simulink library "xpcseriallib"  (Simulink 7.7)
settings: Solver=FixedStepDiscrete  StartTime=0.0  StopTime=inf  RelTol=1e-3
undefined symbols (not defined in the file or in its folder): baddr1, baddr2, mbaseserialbinmask, mbaseserialmask, mdiamondemeraldfifomask, mdiamondemeraldmask, mmodemcontrol, mqua2mask, mquafifomask, mquamask, mrs232
libraries: xpcseriallib x614, xpclib x16, simulink x12
(part 4 of 7)

== system xpcseriallib/Diamond/Emerald-MM /Diamond Emerald-MM ==
  "Enable TX " : S-Function  FunctionName=sertxenableemeraldmm  Parameters=addr  EnableBusSupport=off  mask(Enable TX Int){addr=-1}
      mask prompts: addr "Base address:"
      mask help:
      | Diamond Emerald
      | Enable TX Interrupt
      mask init:
      | addr = hex2dec( addr(3:end) );
      mask Help: helpview(fullfile(docroot, 'mapfiles', 'xpc.map'), 'Baseboard_Enable_Int')
      mask Display:
      | disp('Diamond\nEmerald-MM\nEnable TX int');
      | port_label('input', 1, 'E');
  Filter Int Reason : S-Function  FunctionName=filterserint  Parameters=port, value  EnableBusSupport=off  mask(Interrupt Source Filter){port=1, value=Receive data}
      mask prompts: value "Filter value:"
      mask help:
      | Diamond Emerald-MM
      | Interrupt Source Filter
      mask Help: helpview(fullfile(docroot, 'mapfiles', 'xpc.map'), 'Baseboard_Filter_Ints')
      mask StyleString: popup(1|2|3|4),popup(Receive data|Transmitter empty|Modem status change)
      mask Display:
      | disp('Diamond\nEmerald\nFilter');
      | port_label('input', 1, 'S' );
      | port_label('output', 1, 'E' );
  Read HW FIFO : S-Function  FunctionName=serreademeraldmm  Parameters=addr, flush  EnableBusSupport=off  mask(Read Data Port){flush=on, addr=0}
      mask prompts: flush "Flush HW FIFO on startup"; addr "Base address:"
      mask help:
      | Diamond Emerald-MM
      | Read Data Port
      mask init:
      | addr = hex2dec( addr(3:end) );
      mask Help: helpview(fullfile(docroot, 'mapfiles', 'xpc.map'), 'Baseboard_Read_HW')
      mask Display:
      | disp('Diamond\nEmerald-MM\nRead Data Port');
      | port_label('input', 1, 'E');
      | port_label('output', 1, 'D');
  Read Int Status : S-Function  FunctionName=iqueryemeraldmm  Parameters=addr1, addr2, addr3, addr4, intstat  EnableBusSupport=off  mask(Interrupt Query){addr1=0, addr2=0, addr3=0, addr4=0, intstat=0}
      mask prompts: addr1 "First port address:"; addr2 "Second port address:"; addr3 "Third port address:"; addr4 "Fourth port address:"; intstat "Interrupt status address"
      mask help:
      | Diamond Emerald-MM
      | Interrupt Query
      mask init:
      | addr1 = hex2dec( addr1(3:end) );
      | addr2 = hex2dec( addr2(3:end) );
      | addr3 = hex2dec( addr3(3:end) );
      | addr4 = hex2dec( addr4(3:end) );
      | intstat = hex2dec( intstat(3:end) );
      mask Help: helpview(fullfile(docroot, 'mapfiles', 'xpc.map'), 'Baseboard_Interrupt_Query')
      mask Display:
      | disp('Diamond\nEmerald-MM\nInt Status');
      | port_label('output', 1, 'S' );
  Setup : S-Function  FunctionName=sersetupemeraldmm  Parameters=addr, baud, width, nstop, parity, fmode, ctsmode, rlevel  EnableBusSupport=off  mask(setup){baud=115200  (HS 460800), width=8, nstop=1, parity=None, fmode=16 deep, rlevel=half full, ctsmode=on, addr=0}
      mask prompts: baud "Baud rate:"; width "Number of data bits:"; nstop "Number of stop bits:"; fmode "FIFO mode:"; rlevel "Receive trigger level:"; ctsmode "Enable auto RTS/CTS"; addr "Base address:"
      mask help:
      | Diamond Emerald-MM
      | Serial
      | Setup
      mask init:
      | addr = hex2dec( addr(3:end) );
      mask Help: helpview(fullfile(docroot, 'mapfiles', 'xpc.map'), 'Baseboard_Setup')
      mask StyleString: popup(115200  (HS 460800)|57600   (HS 230400)|38400   (HS 153600)|28800   (HS 115200)|19200   (HS 76800)|14400   (HS 57600)|9600    (HS 38400)|4800    (HS 19200)|2400    (HS 9600)|1200    (HS 4800)|600     (HS 2400)|300     (HS 1200)|150     (HS 600)|110     (HS 440)|75      (HS 300)|27.5    (HS 110)),popup(5|6|7|8),popup(1|2),popup(None|Even|Odd|Mark|Space),popup(64 deep|16 deep|1 deep),popup(1|quarter full|half full|almost full),checkbox,edit
      mask Display: disp('Diamond\nEmerald-MM\nSetup');
  Write HW FIFO : S-Function  FunctionName=serwriteemeraldmm  Parameters=addr  EnableBusSupport=off  mask(Write Data Port){addr=-1}
      mask prompts: addr "Base address:"
      mask help:
      | Diamond Emerald-MM
      | Write Data Port
      mask init:
      | addr = hex2dec( addr(3:end) );
      mask Help: helpview(fullfile(docroot, 'mapfiles', 'xpc.map'), 'Baseboard_Write_HW')
      mask Display:
      | disp('Diamond\nEmerald-MM\nWrite Data Port');
      | port_label('input', 1, 'D');
      | port_label('input', 2, 'E');

== system xpcseriallib/Diamond/Emerald-MM /Diamond Emerald-MM Serial ==
  In1 : Inport
  In2 : Inport  Port=2
  In3 : Inport  Port=3
  In4 : Inport  Port=4
  Enable TX 1 : xpcseriallib/Diamond/Emerald-MM /Diamond Emerald-MM/Enable TX   addr=baddr1
  Enable TX 2 : xpcseriallib/Diamond/Emerald-MM /Diamond Emerald-MM/Enable TX   addr=baddr2
  Enable TX 3 : xpcseriallib/Diamond/Emerald-MM /Diamond Emerald-MM/Enable TX   addr=baddr3
  Enable TX 4 : xpcseriallib/Diamond/Emerald-MM /Diamond Emerald-MM/Enable TX   addr=baddr4
  FIFO read {1..4} (4 alike) : xpcseriallib/FIFO read   maxsize=1024  minsize=1  usedelimiter=on  delimiter=13  outputtype=count+16 bit uint  enable=off  enableout=off  sampletime=-1
  FIFO write 1 : xpcseriallib/FIFO write   size=1024  inputtype=8 bit uint null terminated  present=on  sampletime=-1  id=XMT channel 1, IRQ 7
  FIFO write 2 : xpcseriallib/FIFO write   size=1024  inputtype=8 bit uint null terminated  present=on  sampletime=-1  id=XMT channel 2, IRQ 7
  FIFO write 3 : xpcseriallib/FIFO write   size=1024  inputtype=8 bit uint null terminated  present=on  sampletime=-1  id=XMT channel 3, IRQ 7
  FIFO write 4 : xpcseriallib/FIFO write   size=1024  inputtype=8 bit uint null terminated  present=on  sampletime=-1  id=XMT channel 4, IRQ 7
  IRQ Source : xpclib/Asynchronous Event/IRQ Source  irqNo=7  preempt=10  b_type=None/Other  slot=-1
  RS232 ISR : Subsystem  TreatAsAtomicUnit=on  mask(RS232 ISR){addr1=baddr1, addr2=baddr2, addr3=baddr3, addr4=baddr4, intstat=istat}
      mask prompts: addr1 "First channel address:"; addr2 "Second channel address:"; addr3 "Third channel address:"; addr4 "Fourth channel address:"; intstat "Status register address:"
      mask help:
      | Baseboard Serial
      | Interrupt Service Routine
      mask init:
      | baddr1 = addr1;
      | baddr2 = addr2;
      | baddr3 = addr3;
      | baddr4 = addr4;
      | istat = intstat;
      mask Display:
      | disp('Diamond\nEmerald\nSerial\nISR');
      | port_label('input', 1, 'XMT1');
      | port_label('input', 2, 'XMT2');
      | port_label('input', 3, 'XMT3');
      | port_label('input', 4, 'XMT4');
      | port_label('output', 1, 'RCV1');
      | port_label('output', 2, 'RCV2');
      | port_label('output', 3, 'RCV3');
      | port_label('output', 4, 'RCV4');
  Rate Transition{,1..7} (8 alike) : RateTransition  Integrity=off  Deterministic=off
  Setup1 : xpcseriallib/Diamond/Emerald-MM /Diamond Emerald-MM/Setup  baud="115200  (HS 460800)"  width=8  nstop=1  parity=None  fmode=16 deep  rlevel=half full  ctsmode=on  addr=baddr1
  Setup2 : xpcseriallib/Diamond/Emerald-MM /Diamond Emerald-MM/Setup  baud="115200  (HS 460800)"  width=8  nstop=1  parity=None  fmode=16 deep  rlevel=half full  ctsmode=on  addr=baddr2
  Setup3 : xpcseriallib/Diamond/Emerald-MM /Diamond Emerald-MM/Setup  baud="115200  (HS 460800)"  width=8  nstop=1  parity=None  fmode=16 deep  rlevel=half full  ctsmode=on  addr=baddr3
  Setup4 : xpcseriallib/Diamond/Emerald-MM /Diamond Emerald-MM/Setup  baud="115200  (HS 460800)"  width=8  nstop=1  parity=None  fmode=16 deep  rlevel=half full  ctsmode=on  addr=baddr4
  Out1 : Outport
  Out2 : Outport  Port=2
  Out3 : Outport  Port=3
  Out4 : Outport  Port=4
  wires:
  FIFO write 1/2 -> Enable TX 1/1
  IRQ Source/1 -> RS232 ISR/Trigger
  Rate Transition/1 -> RS232 ISR/1(Xmt 1)
  FIFO write 1/1 -> Rate Transition/1
  In1/1 -> FIFO write 1/1
  FIFO write 2/1 -> Rate Transition2/1
  In2/1 -> FIFO write 2/1
  Rate Transition1/1 -> FIFO read 1/1
  FIFO read 1/1 -> Out1/1
  Rate Transition3/1 -> FIFO read 2/1
  FIFO read 2/1 -> Out2/1
  RS232 ISR/1(Recv 1) -> Rate Transition1/1
  RS232 ISR/2(Recv 2) -> Rate Transition3/1
  Rate Transition2/1 -> RS232 ISR/2(Xmt 2)
  In4/1 -> FIFO write 4/1
  In3/1 -> FIFO write 3/1
  FIFO read 3/1 -> Out3/1
  FIFO read 4/1 -> Out4/1
  Rate Transition5/1 -> FIFO read 3/1
  Rate Transition7/1 -> FIFO read 4/1
  FIFO write 4/1 -> Rate Transition6/1
  FIFO write 3/1 -> Rate Transition4/1
  Rate Transition4/1 -> RS232 ISR/3(Xmt 3)
  Rate Transition6/1 -> RS232 ISR/4(Xmt 4)
  RS232 ISR/3(Recv 3) -> Rate Transition5/1
  RS232 ISR/4(Recv 4) -> Rate Transition7/1
  FIFO write 2/2 -> Enable TX 2/1
  FIFO write 3/2 -> Enable TX 3/1
  FIFO write 4/2 -> Enable TX 4/1

== system xpcseriallib/Diamond/Emerald-MM /Diamond Emerald-MM Serial F ==
  In1 : Inport
  In2 : Inport  Port=2
  In3 : Inport  Port=3
  In4 : Inport  Port=4
  Enable TX 1 : xpcseriallib/Diamond/Emerald-MM /Diamond Emerald-MM/Enable TX   addr=baddr1
  Enable TX 2 : xpcseriallib/Diamond/Emerald-MM /Diamond Emerald-MM/Enable TX   addr=baddr2
  Enable TX 3 : xpcseriallib/Diamond/Emerald-MM /Diamond Emerald-MM/Enable TX   addr=baddr3
  Enable TX 4 : xpcseriallib/Diamond/Emerald-MM /Diamond Emerald-MM/Enable TX   addr=baddr4
  FIFO write 1 : xpcseriallib/FIFO write   size=1024  inputtype=8 bit uint null terminated  present=on  sampletime=-1  id=XMT channel 1, IRQ 7
  FIFO write 2 : xpcseriallib/FIFO write   size=1024  inputtype=8 bit uint null terminated  present=on  sampletime=-1  id=XMT channel 2, IRQ 7
  FIFO write 3 : xpcseriallib/FIFO write   size=1024  inputtype=8 bit uint null terminated  present=on  sampletime=-1  id=XMT channel 3, IRQ 7
  FIFO write 4 : xpcseriallib/FIFO write   size=1024  inputtype=8 bit uint null terminated  present=on  sampletime=-1  id=XMT channel 4, IRQ 7
  IRQ Source : xpclib/Asynchronous Event/IRQ Source  irqNo=7  preempt=10  b_type=None/Other  slot=-1
  RS232 ISR : Subsystem  TreatAsAtomicUnit=on  mask(RS232 ISR){addr1=baddr1, addr2=baddr2, addr3=baddr3, addr4=baddr4, intstat=istat}
      mask prompts: addr1 "First channel address:"; addr2 "Second channel address:"; addr3 "Third channel address:"; addr4 "Fourth channel address:"; intstat "Status register address:"
      mask help:
      | Baseboard Serial
      | Interrupt Service Routine
      mask init:
      | baddr1 = addr1;
      | baddr2 = addr2;
      | baddr3 = addr3;
      | baddr4 = addr4;
      | istat = intstat;
      mask Display:
      | disp('Diamond\nEmerald\nSerial\nISR');
      | port_label('input', 1, 'XMT1');
      | port_label('input', 2, 'XMT2');
      | port_label('input', 3, 'XMT3');
      | port_label('input', 4, 'XMT4');
      | port_label('output', 1, 'RCV1');
      | port_label('output', 2, 'RCV2');
      | port_label('output', 3, 'RCV3');
      | port_label('output', 4, 'RCV4');
  Rate Transition{,2,4,6} (4 alike) : RateTransition  Integrity=off  Deterministic=off
  Rate Transition{1,3,5,7} (4 alike) : RateTransition  Integrity=off  Deterministic=off  OutPortSampleTime=0
  Setup1 : xpcseriallib/Diamond/Emerald-MM /Diamond Emerald-MM/Setup  baud="115200  (HS 460800)"  width=8  nstop=1  parity=None  fmode=16 deep  rlevel=half full  ctsmode=on  addr=baddr1
  Setup2 : xpcseriallib/Diamond/Emerald-MM /Diamond Emerald-MM/Setup  baud="115200  (HS 460800)"  width=8  nstop=1  parity=None  fmode=16 deep  rlevel=half full  ctsmode=on  addr=baddr2
  Setup3 : xpcseriallib/Diamond/Emerald-MM /Diamond Emerald-MM/Setup  baud="115200  (HS 460800)"  width=8  nstop=1  parity=None  fmode=16 deep  rlevel=half full  ctsmode=on  addr=baddr3
  Setup4 : xpcseriallib/Diamond/Emerald-MM /Diamond Emerald-MM/Setup  baud="115200  (HS 460800)"  width=8  nstop=1  parity=None  fmode=16 deep  rlevel=half full  ctsmode=on  addr=baddr4
  Out1 : Outport
  Out2 : Outport  Port=2
  Out3 : Outport  Port=3
  Out4 : Outport  Port=4
  wires:
  FIFO write 1/2 -> Enable TX 1/1
  IRQ Source/1 -> RS232 ISR/Trigger
  Rate Transition/1 -> RS232 ISR/1(Xmt 1)
  FIFO write 1/1 -> Rate Transition/1
  In1/1 -> FIFO write 1/1
  FIFO write 2/1 -> Rate Transition2/1
  In2/1 -> FIFO write 2/1
  Rate Transition1/1 -> Out1/1
  Rate Transition3/1 -> Out2/1
  RS232 ISR/1(Recv 1) -> Rate Transition1/1
  RS232 ISR/2(Recv 2) -> Rate Transition3/1
  Rate Transition2/1 -> RS232 ISR/2(Xmt 2)
  In4/1 -> FIFO write 4/1
  In3/1 -> FIFO write 3/1
  Rate Transition5/1 -> Out3/1
  Rate Transition7/1 -> Out4/1
  FIFO write 4/1 -> Rate Transition6/1
  FIFO write 3/1 -> Rate Transition4/1
  Rate Transition4/1 -> RS232 ISR/3(Xmt 3)
  Rate Transition6/1 -> RS232 ISR/4(Xmt 4)
  RS232 ISR/3(Recv 3) -> Rate Transition5/1
  RS232 ISR/4(Recv 4) -> Rate Transition7/1
  FIFO write 2/2 -> Enable TX 2/1
  FIFO write 3/2 -> Enable TX 3/1
  FIFO write 4/2 -> Enable TX 4/1

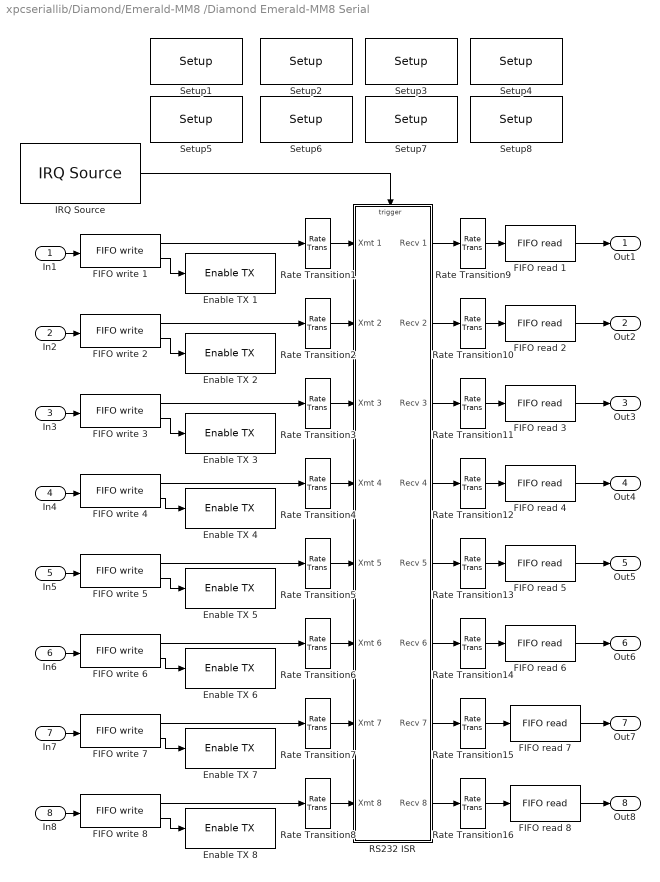
== system xpcseriallib/Diamond/Emerald-MM8 /Diamond Emerald-MM8 Serial ==
  In1 : Inport
  In2 : Inport  Port=2
  In3 : Inport  Port=3
  In4 : Inport  Port=4
  In5 : Inport  Port=5
  In6 : Inport  Port=6
  In7 : Inport  Port=7
  In8 : Inport  Port=8
  Enable TX 1 : xpcseriallib/Diamond/Emerald-MM8 /Diamond Emerald-MM8 /Enable TX   addr=baddr1
  Enable TX 2 : xpcseriallib/Diamond/Emerald-MM8 /Diamond Emerald-MM8 /Enable TX   addr=baddr2
  Enable TX 3 : xpcseriallib/Diamond/Emerald-MM8 /Diamond Emerald-MM8 /Enable TX   addr=baddr3
  Enable TX 4 : xpcseriallib/Diamond/Emerald-MM8 /Diamond Emerald-MM8 /Enable TX   addr=baddr4
  Enable TX 5 : xpcseriallib/Diamond/Emerald-MM8 /Diamond Emerald-MM8 /Enable TX   addr=baddr5
  Enable TX 6 : xpcseriallib/Diamond/Emerald-MM8 /Diamond Emerald-MM8 /Enable TX   addr=baddr6
  Enable TX 7 : xpcseriallib/Diamond/Emerald-MM8 /Diamond Emerald-MM8 /Enable TX   addr=baddr7
  Enable TX 8 : xpcseriallib/Diamond/Emerald-MM8 /Diamond Emerald-MM8 /Enable TX   addr=baddr8
  FIFO read {1..8} (8 alike) : xpcseriallib/FIFO read   maxsize=1024  minsize=1  usedelimiter=on  delimiter=13  outputtype=count+16 bit uint  enable=off  enableout=off  sampletime=-1
  FIFO write 1 : xpcseriallib/FIFO write   size=1024  inputtype=8 bit uint null terminated  present=on  sampletime=-1  id=XMT channel 1, IRQ 5
  FIFO write 2 : xpcseriallib/FIFO write   size=1024  inputtype=8 bit uint null terminated  present=on  sampletime=-1  id=XMT channel 2, IRQ 5
  FIFO write 3 : xpcseriallib/FIFO write   size=1024  inputtype=8 bit uint null terminated  present=on  sampletime=-1  id=XMT channel 3, IRQ 5
  FIFO write 4 : xpcseriallib/FIFO write   size=1024  inputtype=8 bit uint null terminated  present=on  sampletime=-1  id=XMT channel 4, IRQ 5
  FIFO write 5 : xpcseriallib/FIFO write   size=1024  inputtype=8 bit uint null terminated  present=on  sampletime=-1  id=XMT channel 5, IRQ 5
  FIFO write 6 : xpcseriallib/FIFO write   size=1024  inputtype=8 bit uint null terminated  present=on  sampletime=-1  id=XMT channel 6, IRQ 5
  FIFO write 7 : xpcseriallib/FIFO write   size=1024  inputtype=8 bit uint null terminated  present=on  sampletime=-1  id=XMT channel 7, IRQ 5
  FIFO write 8 : xpcseriallib/FIFO write   size=1024  inputtype=8 bit uint null terminated  present=on  sampletime=-1  id=XMT channel 8, IRQ 5
  IRQ Source : xpclib/Asynchronous Event/IRQ Source  irqNo=5  preempt=10  b_type=None/Other  slot=-1
  RS232 ISR : Subsystem  TreatAsAtomicUnit=on  mask(RS232 ISR){addr1=baddr1, addr2=baddr2, addr3=baddr3, addr4=baddr4, intstat=istat}
      mask prompts: addr1 "First channel address:"; addr2 "Second channel address:"; addr3 "Third channel address:"; addr4 "Fourth channel address:"; intstat "Status register address:"
      mask help:
      | Baseboard Serial
      | Interrupt Service Routine
      mask init:
      | baddr1 = addr1;
      | baddr2 = addr2;
      | baddr3 = addr3;
      | baddr4 = addr4;
      | istat = intstat;
      mask Display:
      | disp('Diamond\nEmerald\nSerial\nISR');
      | port_label('input', 1, 'XMT1');
      | port_label('input', 2, 'XMT2');
      | port_label('input', 3, 'XMT3');
      | port_label('input', 4, 'XMT4');
      | port_label('input', 5, 'XMT5');
      | port_label('input', 6, 'XMT6');
      | port_label('input', 7, 'XMT7');
      | port_label('input', 8, 'XMT8');
      | port_label('output', 1, 'RCV1');
      | port_label('output', 2, 'RCV2');
      | port_label('output', 3, 'RCV3');
      | port_label('output', 4, 'RCV4');
      | port_label('output', 5, 'RCV5');
      | port_label('output', 6, 'RCV6');
      | port_label('output', 7, 'RCV7');
      | port_label('output', 8, 'RCV8');
  Rate Transition{1..16} (16 alike) : RateTransition  Integrity=off  Deterministic=off
  Setup1 : xpcseriallib/Diamond/Emerald-MM8 /Diamond Emerald-MM8 /Setup  baud=115200  width=8  nstop=1  parity=None  fmode=16 deep  rlevel=1  ctsmode=on  addr=baddr1  irq=irqnum
  Setup2 : xpcseriallib/Diamond/Emerald-MM8 /Diamond Emerald-MM8 /Setup  baud=115200  width=8  nstop=1  parity=None  fmode=16 deep  rlevel=1  ctsmode=on  addr=baddr2  irq=irqnum
  Setup3 : xpcseriallib/Diamond/Emerald-MM8 /Diamond Emerald-MM8 /Setup  baud=115200  width=8  nstop=1  parity=None  fmode=16 deep  rlevel=1  ctsmode=on  addr=baddr3  irq=irqnum
  Setup4 : xpcseriallib/Diamond/Emerald-MM8 /Diamond Emerald-MM8 /Setup  baud=115200  width=8  nstop=1  parity=None  fmode=16 deep  rlevel=1  ctsmode=on  addr=baddr4  irq=irqnum
  Setup5 : xpcseriallib/Diamond/Emerald-MM8 /Diamond Emerald-MM8 /Setup  baud=115200  width=8  nstop=1  parity=None  fmode=16 deep  rlevel=1  ctsmode=on  addr=baddr5  irq=irqnum
  Setup6 : xpcseriallib/Diamond/Emerald-MM8 /Diamond Emerald-MM8 /Setup  baud=115200  width=8  nstop=1  parity=None  fmode=16 deep  rlevel=1  ctsmode=on  addr=baddr6  irq=irqnum
  Setup7 : xpcseriallib/Diamond/Emerald-MM8 /Diamond Emerald-MM8 /Setup  baud=115200  width=8  nstop=1  parity=None  fmode=16 deep  rlevel=1  ctsmode=on  addr=baddr7  irq=irqnum
  Setup8 : xpcseriallib/Diamond/Emerald-MM8 /Diamond Emerald-MM8 /Setup  baud=115200  width=8  nstop=1  parity=None  fmode=16 deep  rlevel=1  ctsmode=on  addr=baddr8  irq=irqnum
  Out1 : Outport
  Out2 : Outport  Port=2
  Out3 : Outport  Port=3
  Out4 : Outport  Port=4
  Out5 : Outport  Port=5
  Out6 : Outport  Port=6
  Out7 : Outport  Port=7
  Out8 : Outport  Port=8
  wires:
  IRQ Source/1 -> RS232 ISR/Trigger
  Rate Transition1/1 -> RS232 ISR/1(Xmt 1)
  FIFO write 1/1 -> Rate Transition1/1
  In1/1 -> FIFO write 1/1
  In2/1 -> FIFO write 2/1
  Rate Transition9/1 -> FIFO read 1/1
  FIFO read 1/1 -> Out1/1
  Rate Transition10/1 -> FIFO read 2/1
  FIFO read 2/1 -> Out2/1
  RS232 ISR/1(Recv 1) -> Rate Transition9/1
  RS232 ISR/2(Recv 2) -> Rate Transition10/1
  Rate Transition2/1 -> RS232 ISR/2(Xmt 2)
  In4/1 -> FIFO write 4/1
  In3/1 -> FIFO write 3/1
  FIFO read 3/1 -> Out3/1
  FIFO read 4/1 -> Out4/1
  Rate Transition11/1 -> FIFO read 3/1
  Rate Transition12/1 -> FIFO read 4/1
  FIFO write 4/1 -> Rate Transition4/1
  FIFO write 3/1 -> Rate Transition3/1
  Rate Transition3/1 -> RS232 ISR/3(Xmt 3)
  Rate Transition4/1 -> RS232 ISR/4(Xmt 4)
  RS232 ISR/3(Recv 3) -> Rate Transition11/1
  RS232 ISR/4(Recv 4) -> Rate Transition12/1
  FIFO write 1/2 -> Enable TX 1/1
  FIFO write 2/2 -> Enable TX 2/1
  FIFO write 3/2 -> Enable TX 3/1
  FIFO write 4/2 -> Enable TX 4/1
  In5/1 -> FIFO write 5/1
  FIFO write 5/1 -> Rate Transition5/1
  FIFO write 5/2 -> Enable TX 5/1
  In6/1 -> FIFO write 6/1
  FIFO write 6/1 -> Rate Transition6/1
  FIFO write 6/2 -> Enable TX 6/1
  In7/1 -> FIFO write 7/1
  FIFO write 7/1 -> Rate Transition7/1
  FIFO write 7/2 -> Enable TX 7/1
  In8/1 -> FIFO write 8/1
  FIFO write 8/1 -> Rate Transition8/1
  FIFO write 8/2 -> Enable TX 8/1
  Rate Transition13/1 -> FIFO read 5/1
  FIFO read 5/1 -> Out5/1
  Rate Transition14/1 -> FIFO read 6/1
  FIFO read 6/1 -> Out6/1
  Rate Transition15/1 -> FIFO read 7/1
  FIFO read 7/1 -> Out7/1
  Rate Transition16/1 -> FIFO read 8/1
  FIFO read 8/1 -> Out8/1
  Rate Transition5/1 -> RS232 ISR/5(Xmt 5)
  Rate Transition6/1 -> RS232 ISR/6(Xmt 6)
  Rate Transition7/1 -> RS232 ISR/7(Xmt 7)
  Rate Transition8/1 -> RS232 ISR/8(Xmt 8)
  RS232 ISR/5(Recv 5) -> Rate Transition13/1
  RS232 ISR/6(Recv 6) -> Rate Transition14/1
  RS232 ISR/7(Recv 7) -> Rate Transition15/1
  RS232 ISR/8(Recv 8) -> Rate Transition16/1
  FIFO write 2/1 -> Rate Transition2/1

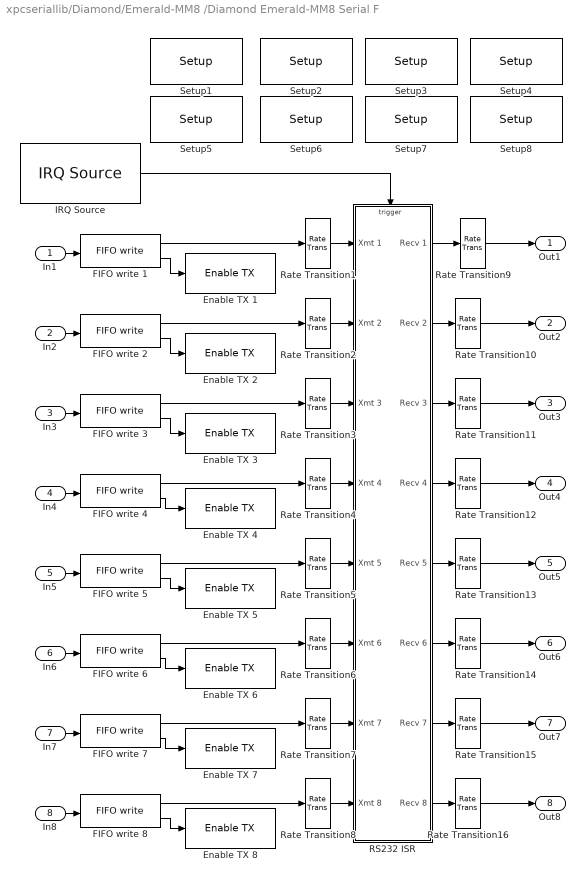
== system xpcseriallib/Diamond/Emerald-MM8 /Diamond Emerald-MM8 Serial F ==
  In1 : Inport
  In2 : Inport  Port=2
  In3 : Inport  Port=3
  In4 : Inport  Port=4
  In5 : Inport  Port=5
  In6 : Inport  Port=6
  In7 : Inport  Port=7
  In8 : Inport  Port=8
  Enable TX 1 : xpcseriallib/Diamond/Emerald-MM8 /Diamond Emerald-MM8 /Enable TX   addr=baddr1
  Enable TX 2 : xpcseriallib/Diamond/Emerald-MM8 /Diamond Emerald-MM8 /Enable TX   addr=baddr2
  Enable TX 3 : xpcseriallib/Diamond/Emerald-MM8 /Diamond Emerald-MM8 /Enable TX   addr=baddr3
  Enable TX 4 : xpcseriallib/Diamond/Emerald-MM8 /Diamond Emerald-MM8 /Enable TX   addr=baddr4
  Enable TX 5 : xpcseriallib/Diamond/Emerald-MM8 /Diamond Emerald-MM8 /Enable TX   addr=baddr5
  Enable TX 6 : xpcseriallib/Diamond/Emerald-MM8 /Diamond Emerald-MM8 /Enable TX   addr=baddr6
  Enable TX 7 : xpcseriallib/Diamond/Emerald-MM8 /Diamond Emerald-MM8 /Enable TX   addr=baddr7
  Enable TX 8 : xpcseriallib/Diamond/Emerald-MM8 /Diamond Emerald-MM8 /Enable TX   addr=baddr8
  FIFO write 1 : xpcseriallib/FIFO write   size=1024  inputtype=8 bit uint null terminated  present=on  sampletime=-1  id=XMT channel 1, IRQ 5
  FIFO write 2 : xpcseriallib/FIFO write   size=1024  inputtype=8 bit uint null terminated  present=on  sampletime=-1  id=XMT channel 2, IRQ 5
  FIFO write 3 : xpcseriallib/FIFO write   size=1024  inputtype=8 bit uint null terminated  present=on  sampletime=-1  id=XMT channel 3, IRQ 5
  FIFO write 4 : xpcseriallib/FIFO write   size=1024  inputtype=8 bit uint null terminated  present=on  sampletime=-1  id=XMT channel 4, IRQ 5
  FIFO write 5 : xpcseriallib/FIFO write   size=1024  inputtype=8 bit uint null terminated  present=on  sampletime=-1  id=XMT channel 5, IRQ 5
  FIFO write 6 : xpcseriallib/FIFO write   size=1024  inputtype=8 bit uint null terminated  present=on  sampletime=-1  id=XMT channel 6, IRQ 5
  FIFO write 7 : xpcseriallib/FIFO write   size=1024  inputtype=8 bit uint null terminated  present=on  sampletime=-1  id=XMT channel 7, IRQ 5
  FIFO write 8 : xpcseriallib/FIFO write   size=1024  inputtype=8 bit uint null terminated  present=on  sampletime=-1  id=XMT channel 8, IRQ 5
  IRQ Source : xpclib/Asynchronous Event/IRQ Source  irqNo=5  preempt=10  b_type=None/Other  slot=-1
  RS232 ISR : Subsystem  TreatAsAtomicUnit=on  mask(RS232 ISR){addr1=baddr1, addr2=baddr2, addr3=baddr3, addr4=baddr4, intstat=istat}
      mask prompts: addr1 "First channel address:"; addr2 "Second channel address:"; addr3 "Third channel address:"; addr4 "Fourth channel address:"; intstat "Status register address:"
      mask help:
      | Baseboard Serial
      | Interrupt Service Routine
      mask init:
      | baddr1 = addr1;
      | baddr2 = addr2;
      | baddr3 = addr3;
      | baddr4 = addr4;
      | istat = intstat;
      mask Display:
      | disp('Diamond\nEmerald\nSerial\nISR');
      | port_label('input', 1, 'XMT1');
      | port_label('input', 2, 'XMT2');
      | port_label('input', 3, 'XMT3');
      | port_label('input', 4, 'XMT4');
      | port_label('input', 5, 'XMT5');
      | port_label('input', 6, 'XMT6');
      | port_label('input', 7, 'XMT7');
      | port_label('input', 8, 'XMT8');
      | port_label('output', 1, 'RCV1');
      | port_label('output', 2, 'RCV2');
      | port_label('output', 3, 'RCV3');
      | port_label('output', 4, 'RCV4');
      | port_label('output', 5, 'RCV5');
      | port_label('output', 6, 'RCV6');
      | port_label('output', 7, 'RCV7');
      | port_label('output', 8, 'RCV8');
  Rate Transition{1..8} (8 alike) : RateTransition  Integrity=off  Deterministic=off
  Rate Transition{9..16} (8 alike) : RateTransition  Integrity=off  Deterministic=off  OutPortSampleTime=0
  Setup1 : xpcseriallib/Diamond/Emerald-MM8 /Diamond Emerald-MM8 /Setup  baud=115200  width=8  nstop=1  parity=None  fmode=16 deep  rlevel=1  ctsmode=on  addr=baddr1  irq=irqnum
  Setup2 : xpcseriallib/Diamond/Emerald-MM8 /Diamond Emerald-MM8 /Setup  baud=115200  width=8  nstop=1  parity=None  fmode=16 deep  rlevel=1  ctsmode=on  addr=baddr2  irq=irqnum
  Setup3 : xpcseriallib/Diamond/Emerald-MM8 /Diamond Emerald-MM8 /Setup  baud=115200  width=8  nstop=1  parity=None  fmode=16 deep  rlevel=1  ctsmode=on  addr=baddr3  irq=irqnum
  Setup4 : xpcseriallib/Diamond/Emerald-MM8 /Diamond Emerald-MM8 /Setup  baud=115200  width=8  nstop=1  parity=None  fmode=16 deep  rlevel=1  ctsmode=on  addr=baddr4  irq=irqnum
  Setup5 : xpcseriallib/Diamond/Emerald-MM8 /Diamond Emerald-MM8 /Setup  baud=115200  width=8  nstop=1  parity=None  fmode=16 deep  rlevel=1  ctsmode=on  addr=baddr5  irq=irqnum
  Setup6 : xpcseriallib/Diamond/Emerald-MM8 /Diamond Emerald-MM8 /Setup  baud=115200  width=8  nstop=1  parity=None  fmode=16 deep  rlevel=1  ctsmode=on  addr=baddr6  irq=irqnum
  Setup7 : xpcseriallib/Diamond/Emerald-MM8 /Diamond Emerald-MM8 /Setup  baud=115200  width=8  nstop=1  parity=None  fmode=16 deep  rlevel=1  ctsmode=on  addr=baddr7  irq=irqnum
  Setup8 : xpcseriallib/Diamond/Emerald-MM8 /Diamond Emerald-MM8 /Setup  baud=115200  width=8  nstop=1  parity=None  fmode=16 deep  rlevel=1  ctsmode=on  addr=baddr8  irq=irqnum
  Out1 : Outport
  Out2 : Outport  Port=2
  Out3 : Outport  Port=3
  Out4 : Outport  Port=4
  Out5 : Outport  Port=5
  Out6 : Outport  Port=6
  Out7 : Outport  Port=7
  Out8 : Outport  Port=8
  wires:
  IRQ Source/1 -> RS232 ISR/Trigger
  Rate Transition1/1 -> RS232 ISR/1(Xmt 1)
  FIFO write 1/1 -> Rate Transition1/1
  In1/1 -> FIFO write 1/1
  In2/1 -> FIFO write 2/1
  Rate Transition9/1 -> Out1/1
  Rate Transition10/1 -> Out2/1
  RS232 ISR/1(Recv 1) -> Rate Transition9/1
  RS232 ISR/2(Recv 2) -> Rate Transition10/1
  Rate Transition2/1 -> RS232 ISR/2(Xmt 2)
  In4/1 -> FIFO write 4/1
  In3/1 -> FIFO write 3/1
  Rate Transition11/1 -> Out3/1
  Rate Transition12/1 -> Out4/1
  FIFO write 4/1 -> Rate Transition4/1
  FIFO write 3/1 -> Rate Transition3/1
  Rate Transition3/1 -> RS232 ISR/3(Xmt 3)
  Rate Transition4/1 -> RS232 ISR/4(Xmt 4)
  RS232 ISR/3(Recv 3) -> Rate Transition11/1
  RS232 ISR/4(Recv 4) -> Rate Transition12/1
  FIFO write 1/2 -> Enable TX 1/1
  FIFO write 2/2 -> Enable TX 2/1
  FIFO write 3/2 -> Enable TX 3/1
  FIFO write 4/2 -> Enable TX 4/1
  In5/1 -> FIFO write 5/1
  FIFO write 5/1 -> Rate Transition5/1
  FIFO write 5/2 -> Enable TX 5/1
  In6/1 -> FIFO write 6/1
  FIFO write 6/1 -> Rate Transition6/1
  FIFO write 6/2 -> Enable TX 6/1
  In7/1 -> FIFO write 7/1
  FIFO write 7/1 -> Rate Transition7/1
  FIFO write 7/2 -> Enable TX 7/1
  In8/1 -> FIFO write 8/1
  FIFO write 8/1 -> Rate Transition8/1
  FIFO write 8/2 -> Enable TX 8/1
  Rate Transition13/1 -> Out5/1
  Rate Transition14/1 -> Out6/1
  Rate Transition15/1 -> Out7/1
  Rate Transition16/1 -> Out8/1
  Rate Transition5/1 -> RS232 ISR/5(Xmt 5)
  Rate Transition6/1 -> RS232 ISR/6(Xmt 6)
  Rate Transition7/1 -> RS232 ISR/7(Xmt 7)
  Rate Transition8/1 -> RS232 ISR/8(Xmt 8)
  RS232 ISR/5(Recv 5) -> Rate Transition13/1
  RS232 ISR/6(Recv 6) -> Rate Transition14/1
  RS232 ISR/7(Recv 7) -> Rate Transition15/1
  RS232 ISR/8(Recv 8) -> Rate Transition16/1
  FIFO write 2/1 -> Rate Transition2/1

== system xpcseriallib/Diamond/Emerald-MM8 /Diamond Emerald-MM8  ==
  "Enable TX " : S-Function  FunctionName=sertxenableemeraldmm  Parameters=addr  EnableBusSupport=off  mask(Enable TX Int){addr='0x208'}
      mask prompts: addr "Base address:"
      mask help:
      | Diamond Emerald
      | Enable TX Interrupt
      mask init:
      | addr = hex2dec( addr(3:end) );
      mask Help: helpview(fullfile(docroot, 'mapfiles', 'xpc.map'), 'Baseboard_Enable_Int')
      mask Display:
      | disp('Diamond\nEmerald-MM8\nEnable TX int');
      | port_label('input', 1, 'E');
  Filter Int Reason : S-Function  FunctionName=filterserint  Parameters=port, value  EnableBusSupport=off  mask(Interrupt Source Filter){port=1, value=Receive data}
      mask prompts: value "Filter value:"
      mask help:
      | Diamond Emerald-MM
      | Interrupt Source Filter
      mask Help: helpview(fullfile(docroot, 'mapfiles', 'xpc.map'), 'Baseboard_Filter_Ints')
      mask StyleString: popup(1|2|3|4|5|6|7|8),popup(Receive data|Transmitter empty|Modem status change)
      mask Display:
      | disp('Diamond\nEmerald-MM8\nFilter');
      | port_label('input', 1, 'S' );
      | port_label('output', 1, 'E' );
  Read HW FIFO : S-Function  FunctionName=serreademeraldmm  Parameters=addr, flush  EnableBusSupport=off  mask(Read Data Port){flush=on, addr=0}
      mask prompts: flush "Flush HW FIFO on startup"; addr "Base address:"
      mask help:
      | Diamond Emerald-MM
      | Read Data Port
      mask init:
      | addr = hex2dec( addr(3:end) );
      mask Help: helpview(fullfile(docroot, 'mapfiles', 'xpc.map'), 'Baseboard_Read_HW')
      mask Display:
      | disp('Diamond\nEmerald-MM8\nRead Data Port');
      | port_label('input', 1, 'E');
      | port_label('output', 1, 'D');
  Read Int Status : S-Function  FunctionName=iqueryemeraldmm8  Parameters=addr1, addr2, addr3, addr4, addr5, addr6, addr7, addr8, intstat  EnableBusSupport=off  mask(Interrupt Query){addr1=0, addr2=0, addr3=0, addr4=0, addr5=0, addr6=0, addr7=0, addr8=0, intstat=0}
      mask prompts: addr1 "First port address:"; addr2 "Second port address:"; addr3 "Third port address:"; addr4 "Fourth port address:"; addr5 "Fifth port address:"; addr6 "Sixth port address:"; addr7 "Seventh port address:"; addr8 "Eighth port address:"; intstat "Interrupt status address"
      mask help:
      | Diamond Emerald-MM8
      | Interrupt Query
      mask init:
      | addr1 = hex2dec( addr1(3:end) );
      | addr2 = hex2dec( addr2(3:end) );
      | addr3 = hex2dec( addr3(3:end) );
      | addr4 = hex2dec( addr4(3:end) );
      | addr5 = hex2dec( addr5(3:end) );
      | addr6 = hex2dec( addr6(3:end) );
      | addr7 = hex2dec( addr7(3:end) );
      | addr8 = hex2dec( addr8(3:end) );
      | intstat = hex2dec( intstat(3:end) );
      mask Help: helpview(fullfile(docroot, 'mapfiles', 'xpc.map'), 'Baseboard_Interrupt_Query')
      mask Display:
      | disp('Diamond\nEmerald-MM8\nInt Status');
      | port_label('output', 1, 'S' );
  Setup : S-Function  FunctionName=sersetupemeraldmm8  Parameters=addr, irq, baud, width, nstop, parity, fmode, ctsmode, rlevel  EnableBusSupport=off  mask(setup){baud=115200, width=8, nstop=1, parity=None, fmode=16 deep, rlevel=half full, ctsmode=on, addr=0, irq=0}
      mask prompts: baud "Baud rate:"; width "Number of data bits:"; nstop "Number of stop bits:"; fmode "FIFO mode:"; rlevel "Receive trigger level:"; ctsmode "Enable auto RTS/CTS"; addr "Base address:"
      mask help:
      | Diamond Emerald-MM
      | Serial
      | Setup
      mask init:
      | addr = hex2dec( addr(3:end) );
      mask Help: helpview(fullfile(docroot, 'mapfiles', 'xpc.map'), 'Baseboard_Setup')
      mask StyleString: popup(115200|57600|38400|19200|9600|4800|2400|1200|600|300|110),popup(5|6|7|8),popup(1|2),popup(None|Even|Odd|Mark|Space),popup(64 deep|16 deep|1 deep),popup(1|quarter full|half full|almost full),checkbox,edit,edit
      mask Display: disp('Diamond\nEmerald-MM8\nSetup');
  Write HW FIFO : S-Function  FunctionName=serwriteemeraldmm  Parameters=addr  EnableBusSupport=off  mask(Write Data Port){addr=-1}
      mask prompts: addr "Base address:"
      mask help:
      | Diamond Emerald-MM
      | Write Data Port
      mask init:
      | addr = hex2dec( addr(3:end) );
      mask Help: helpview(fullfile(docroot, 'mapfiles', 'xpc.map'), 'Baseboard_Write_HW')
      mask Display:
      | disp('Diamond\nEmerald-MM8\nWrite Data Port');
      | port_label('input', 1, 'D');
      | port_label('input', 2, 'E');

== system xpcseriallib/Mainboard/Baseboard Serial/RS232 ISR ==
  Xmt 1 : Inport
  Xmt 2 : Inport  Port=2
  function : TriggerPort  TriggerType=function-call
  Demux : Demux
  Read Int Status FC1 : xpcseriallib/Mainboard/Baseboard Serial Internal  blocks/Read Int Status FC  addr1=baddr1  addr2=baddr2
  Receive 1 : Subsystem  TreatAsAtomicUnit=on
  Receive 2 : Subsystem  TreatAsAtomicUnit=on
  Transmit 1 : Subsystem  TreatAsAtomicUnit=on
  Transmit 2 : Subsystem  TreatAsAtomicUnit=on
  Recv 1 : Outport
  Recv 2 : Outport  Port=2
  wires:
  Read Int Status FC1/2 -> Transmit 2/2(Enable), Transmit 1/2(Enable)
  Demux/2 -> Transmit 1/Trigger
  Demux/3 -> Receive 2/Trigger
  Demux/4 -> Transmit 2/Trigger
  Demux/1 -> Receive 1/Trigger
  Read Int Status FC1/1 -> Demux/1
  Xmt 2/1 -> Transmit 2/1(Xmt 2)
  Receive 2/1(Recv 2) -> Recv 2/1
  Xmt 1/1 -> Transmit 1/1(Xmt 1)
  Receive 1/1(Recv 1) -> Recv 1/1

== system xpcseriallib/Mainboard/Baseboard Serial F/RS232 ISR ==
  Xmt 1 : Inport
  Xmt 2 : Inport  Port=2
  function : TriggerPort  TriggerType=function-call
  Demux : Demux
  Read Int Status FC1 : xpcseriallib/Mainboard/Baseboard Serial Internal  blocks/Read Int Status FC  addr1=baddr1  addr2=baddr2
  Receive 1 : Subsystem  TreatAsAtomicUnit=on
  Receive 2 : Subsystem  TreatAsAtomicUnit=on
  Transmit 1 : Subsystem  TreatAsAtomicUnit=on
  Transmit 2 : Subsystem  TreatAsAtomicUnit=on
  Recv 1 : Outport
  Recv 2 : Outport  Port=2
  wires:
  Receive 1/1(Recv 1) -> Recv 1/1
  Xmt 1/1 -> Transmit 1/1(Xmt 1)
  Receive 2/1(Recv 2) -> Recv 2/1
  Xmt 2/1 -> Transmit 2/1(Xmt 2)
  Read Int Status FC1/1 -> Demux/1
  Demux/1 -> Receive 1/Trigger
  Demux/4 -> Transmit 2/Trigger
  Demux/3 -> Receive 2/Trigger
  Demux/2 -> Transmit 1/Trigger
  Read Int Status FC1/2 -> Transmit 1/2(Enable), Transmit 2/2(Enable)

== system xpcseriallib/Obsolete V 1.0/Asynchronous Mode/Receive  ==
  S-Function : S-Function  FunctionName=rs232_rec  Parameters=port,formatrec,numb,ts  EnableBusSupport=off
  Out1 : Outport
  wires:
  S-Function/1 -> Out1/1

== system xpcseriallib/Obsolete V 1.0/Asynchronous Mode/Send  ==
  In1 : Inport
  S-Function : S-Function  FunctionName=rs232_send  Parameters=port,formatsend,wait,ts  EnableBusSupport=off
  wires:
  In1/1 -> S-Function/1

== system xpcseriallib/Obsolete V 1.0/Synchronous Mode/Send & Receive  ==
  In1 : Inport
  S-Function : S-Function  FunctionName=rs232_sendrec  Parameters=port,formatsend,formatrec,numb,ts  EnableBusSupport=off
  Out1 : Outport
  wires:
  In1/1 -> S-Function/1
  S-Function/1 -> Out1/1

== system xpcseriallib/Quatech/DSCP-200/300/DSCP-200/300 Internal  blocks ==
  "Enable TX " : S-Function  FunctionName=sertxenable  Parameters=slot, port, 8  SFunctionModules='quatechinit'  EnableBusSupport=off  mask(Enable TX Int){port=1, slot=-1}
      mask prompts: slot "PCI slot: (-1 for autosearch)"
      mask help:
      | DSCP-200/300
      | Quatech
      | Enable TX Interrupt
      mask Help: helpview(fullfile(docroot, 'mapfiles', 'xpc.map'), 'Quatech_Enable_Int')
      mask StyleString: popup(1|2),edit
      mask Display:
      | disp('DSCP-200/300\nQuatech\nEnable TX int');
      | port_label('input', 1, 'E');
  Filter Int Reason : S-Function  FunctionName=filterqua  Parameters=port, 8, value  EnableBusSupport=off  mask(Interrupt Source Filter){port=1, value=Receive data}
      mask prompts: value "Filter value:"
      mask help:
      | DSCP-200/300
      | Quatech
      | Interrupt Source Filter
      mask Help: helpview(fullfile(docroot, 'mapfiles', 'xpc.map'), 'Quatech_Filter_Ints')
      mask StyleString: popup(1|2),popup(Receive data|Transmitter empty|Modem status change)
      mask Display:
      | disp('DSCP-200/300\nQuatech\nFilter Int Reason');
      | port_label('input', 1, 'S' );
      | port_label('output', 1, 'E' );
  Int Check : S-Function  FunctionName=intcheckqua  Parameters=slot, irqnum+2, boardtype,  SFunctionModules='quatechinit'  EnableBusSupport=off  mask(interrupt check){slot=-1, irqnum=5}
      mask prompts: slot "PCI slot: (-1 for autosearch)"; irqnum "IRQ Line Number"
      mask help:
      | DSCP-200/300
      | Quatech
      | Interrupt Check
      mask init:
      | boardtype = 8;
      mask Help: helpview(fullfile(docroot, 'mapfiles', 'xpc.map'), 'Quatech_Interrupt_Check')
      mask StyleString: edit,popup(3|4|5|6|7|8|9|10|11|12|13|14|15)
      mask Display: disp('DSCP-200/300\nQuatech\nInterrupt Check');
  Read HW FIFO : S-Function  FunctionName=serreadqua  Parameters=slot, port, 8, flush  SFunctionModules='quatechinit'  EnableBusSupport=off  mask(Read Data Port){port=1, flush=on, slot=-1}
      mask prompts: flush "Flush HW FIFO on startup"; slot "PCI slot: (-1 for autosearch)"
      mask help:
      | DSCP-200/300
      | Quatech
      | Read Data Port
      mask Help: helpview(fullfile(docroot, 'mapfiles', 'xpc.map'), 'Quatech_Read_HW')
      mask StyleString: popup(1|2),checkbox,edit
      mask Display:
      | disp('DSCP-200/300\nQuatech\nRead HW FIFO');
      | port_label('input', 1, 'E');
      | port_label('output', 1, 'D');
  Read Int Status : S-Function  FunctionName=iqueryqua  Parameters=slot, 8  SFunctionModules='quatechinit'  EnableBusSupport=off  mask(Interrupt Query){slot=-1}
      mask prompts: slot "PCI slot: (-1 for autosearch)"
      mask help:
      | DSCP-200/300
      | Quatech
      | Interrupt Query
      mask Help: helpview(fullfile(docroot, 'mapfiles', 'xpc.map'), 'Quatech_Interrupt_Query')
      mask Display:
      | disp('DSCP-200/300\nQuatech\nRead Int Status');
      | port_label('output', 1, 'S' );
  Setup : S-Function  FunctionName=setupqua  Parameters=slot, boardtype, port, baud, width, nstop, parity, fmode, ctsmode, rlevel  SFunctionModules='quatechinit'  EnableBusSupport=off  mask(setup){port=1, baud=115200, width=8, nstop=1, parity=None, fmode=64 deep, rlevel=half full, ctsmode=off, slot=-1}
      mask prompts: baud "Baud rate:"; width "Number of data bits:"; nstop "Number of stop bits:"; fmode "FIFO mode:"; rlevel "Receive trigger level:"; ctsmode "Enable auto RTS/CTS"; slot "PCI slot: (-1 for autosearch)"
      mask help:
      | DSCP-200/300
      | Quatech
      | Setup
      mask init:
      | boardtype = 8;
      mask Help: helpview(fullfile(docroot, 'mapfiles', 'xpc.map'), 'Quatech_Setup')
      mask StyleString: popup(1|2),popup(921600|460800|230400|115200|57600|38400|19200|9600|4800|2400|1200|600|300|110),popup(5|6|7|8),popup(1|2),popup(None|Even|Odd|Mark|Space),popup(64 deep|16 deep|1 deep),popup(1|quarter full|half full|almost full),checkbox,edit
      mask Display: disp('DSCP-200/300\nQuatech\nSetup');
  Write HW FIFO : S-Function  FunctionName=serwritequa  Parameters=slot, port, 8, onxmt  SFunctionModules='quatechinit'  EnableBusSupport=off  mask(Write Data Port){port=1, onxmt=None, slot=-1}
      mask prompts: onxmt "Assert on Transmit:"; slot "PCI slot: (-1 for autosearch)"
      mask help:
      | DSCP-200/300
      | Quatech
      | Write Data Port
      mask Help: helpview(fullfile(docroot, 'mapfiles', 'xpc.map'), 'Quatech_Write_HW')
      mask StyleString: popup(1|2),popup(None|RTS|DTR),edit
      mask Display:
      | disp('DSCP-200/300\nQuatech\nWrite HW FIFO');
      | port_label('input', 1, 'D');
      | port_label('input', 2, 'E');

== system xpcseriallib/Quatech/DSCP-200/300/DSCP-200/300  ==
  In1 : Inport
  In2 : Inport  Port=2
  Enable TX 1 : xpcseriallib/Quatech/DSCP-200//300/DSCP-200//300 Internal  blocks/Enable TX   port=1  slot=brdslot
  Enable TX 2 : xpcseriallib/Quatech/DSCP-200//300/DSCP-200//300 Internal  blocks/Enable TX   port=2  slot=brdslot
  FIFO read 1 : xpcseriallib/FIFO read   maxsize=1024  minsize=1  usedelimiter=on  delimiter=13  outputtype=count+16 bit uint  enable=off  enableout=off  sampletime=-1
  FIFO read 2 : xpcseriallib/FIFO read   maxsize=1024  minsize=1  usedelimiter=on  delimiter=13  outputtype=count+16 bit uint  enable=off  enableout=off  sampletime=-1
  FIFO write 1 : xpcseriallib/FIFO write   size=1024  inputtype=8 bit uint null terminated  present=on  sampletime=-1  id=XMT channel 1, IRQ Auto (PCI only)
  FIFO write 2 : xpcseriallib/FIFO write   size=1024  inputtype=8 bit uint null terminated  present=on  sampletime=-1  id=XMT channel 2, IRQ Auto (PCI only)
  IRQ Source : xpclib/Asynchronous Event/IRQ Source  irqNo=Auto (PCI only)  preempt=10  b_type=Quatech DSCP-200/300  slot=-1
  RS232 ISR : Subsystem  TreatAsAtomicUnit=on  mask(RS232 ISR){slot=brdslot}
      mask help:
      | DSCP-100
      | Quatech
      | Interrupt Service Routine
      mask init:
      | subslot = slot;
      mask Display:
      | disp('DSCP-200/300\nISR');
      | port_label('input', 1, 'XMT1');
      | port_label('input', 2, 'XMT2');
      | port_label('output', 1, 'RCV1');
      | port_label('output', 2, 'RCV2');
  Rate Transition{,1..3} (4 alike) : RateTransition  Integrity=off  Deterministic=off
  Setup1 : xpcseriallib/Quatech/DSCP-200//300/DSCP-200//300 Internal  blocks/Setup  port=1  baud=115200  width=8  nstop=1  parity=None  fmode=64 deep  rlevel=half full  ctsmode=off  slot=brdslot
  Setup2 : xpcseriallib/Quatech/DSCP-200//300/DSCP-200//300 Internal  blocks/Setup  port=2  baud=115200  width=8  nstop=1  parity=None  fmode=64 deep  rlevel=half full  ctsmode=off  slot=brdslot
  Out1 : Outport
  Out2 : Outport  Port=2
  wires:
  Rate Transition3/1 -> FIFO read 2/1
  FIFO write 1/2 -> Enable TX 1/1
  IRQ Source/1 -> RS232 ISR/Trigger
  Rate Transition/1 -> RS232 ISR/1(Xmt 1)
  RS232 ISR/1(Recv 1) -> Rate Transition1/1
  RS232 ISR/2(Recv 2) -> Rate Transition3/1
  FIFO write 1/1 -> Rate Transition/1
  In1/1 -> FIFO write 1/1
  FIFO write 2/1 -> Rate Transition2/1
  In2/1 -> FIFO write 2/1
  Rate Transition1/1 -> FIFO read 1/1
  FIFO read 1/1 -> Out1/1
  FIFO read 2/1 -> Out2/1
  FIFO write 2/2 -> Enable TX 2/1
  Rate Transition2/1 -> RS232 ISR/2(Xmt 2)

== system xpcseriallib/Quatech/DSCP-200/300/DSCP-200/300 F ==
  In1 : Inport
  In2 : Inport  Port=2
  Enable TX 1 : xpcseriallib/Quatech/DSCP-200//300/DSCP-200//300 Internal  blocks/Enable TX   port=1  slot=brdslot
  Enable TX 2 : xpcseriallib/Quatech/DSCP-200//300/DSCP-200//300 Internal  blocks/Enable TX   port=2  slot=brdslot
  FIFO write 1 : xpcseriallib/FIFO write   size=1024  inputtype=8 bit uint null terminated  present=on  sampletime=-1  id=XMT channel 1, IRQ Auto (PCI only)
  FIFO write 2 : xpcseriallib/FIFO write   size=1024  inputtype=8 bit uint null terminated  present=on  sampletime=-1  id=XMT channel 2, IRQ Auto (PCI only)
  IRQ Source : xpclib/Asynchronous Event/IRQ Source  irqNo=Auto (PCI only)  preempt=10  b_type=Quatech DSCP-200/300  slot=-1
  RS232 ISR : Subsystem  TreatAsAtomicUnit=on  mask(RS232 ISR){slot=brdslot}
      mask help:
      | DSCP-100
      | Quatech
      | Interrupt Service Routine
      mask init:
      | subslot = slot;
      mask Display:
      | disp('DSCP-200/300\nISR');
      | port_label('input', 1, 'XMT1');
      | port_label('input', 2, 'XMT2');
      | port_label('output', 1, 'RCV1');
      | port_label('output', 2, 'RCV2');
  Rate Transition : RateTransition  Integrity=off  Deterministic=off
  Rate Transition1 : RateTransition  Integrity=off  Deterministic=off  OutPortSampleTime=0
  Rate Transition2 : RateTransition  Integrity=off  Deterministic=off
  Rate Transition3 : RateTransition  Integrity=off  Deterministic=off  OutPortSampleTime=0
  Setup1 : xpcseriallib/Quatech/DSCP-200//300/DSCP-200//300 Internal  blocks/Setup  port=1  baud=115200  width=8  nstop=1  parity=None  fmode=64 deep  rlevel=half full  ctsmode=off  slot=brdslot
  Setup2 : xpcseriallib/Quatech/DSCP-200//300/DSCP-200//300 Internal  blocks/Setup  port=2  baud=115200  width=8  nstop=1  parity=None  fmode=64 deep  rlevel=half full  ctsmode=off  slot=brdslot
  Out1 : Outport
  Out2 : Outport  Port=2
  wires:
  Rate Transition3/1 -> Out2/1
  FIFO write 1/2 -> Enable TX 1/1
  IRQ Source/1 -> RS232 ISR/Trigger
  Rate Transition/1 -> RS232 ISR/1(Xmt 1)
  RS232 ISR/1(Recv 1) -> Rate Transition1/1
  RS232 ISR/2(Recv 2) -> Rate Transition3/1
  FIFO write 1/1 -> Rate Transition/1
  In1/1 -> FIFO write 1/1
  FIFO write 2/1 -> Rate Transition2/1
  In2/1 -> FIFO write 2/1
  Rate Transition1/1 -> Out1/1
  FIFO write 2/2 -> Enable TX 2/1
  Rate Transition2/1 -> RS232 ISR/2(Xmt 2)
